simulink model "PIDControllerTest"  (R2025b)
settings: Solver=FixedStepAuto  StartTime=0.0  StopTime=inf  FixedStep=.01  RelTol=1e-3
settings Model: Creator=talles  LastModifiedBy=ajax

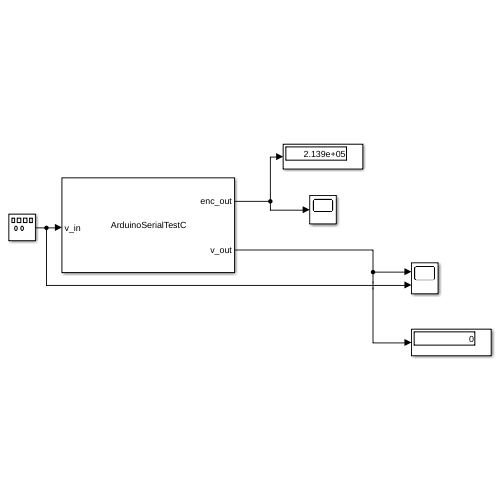
[thumbnail: Simulink's stored preview of the top-level diagram]
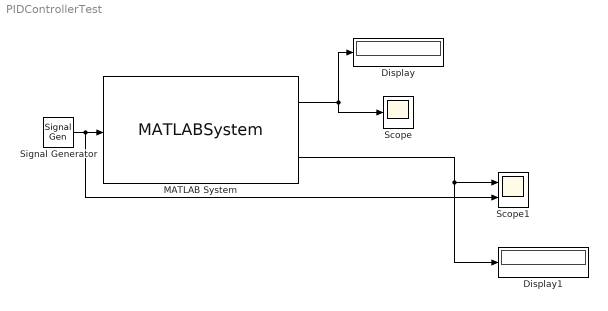
== system PIDControllerTest ==
  Display : Display
  Display1 : Display
  MATLAB System : MATLABSystem  System=ArduinoSerialTestC  COMPort=/dev/ttyACM0  BaudRate=115200  SimulateUsing=Interpreted execution
      mask Type: ArduinoSerialTestC
  Scope : Scope
      settings: ActiveDisplayYMinimum=-1.6860745042674926E+6  ActiveDisplayYMaximum=1.7659047746045869E+6
  Scope1 : Scope  NumInputPorts=2
      settings: ActiveDisplayYMinimum=-6.0034594760493682  ActiveDisplayYMaximum=14.706273819701902
  Signal Generator : SignalGenerator  WaveForm=square  Frequency=.5
  wires:
  MATLAB System/1 -> Display/1, Scope/1
  MATLAB System/2 -> Display1/1, Scope1/1
  Signal Generator/1 -> Scope1/2, MATLAB System/1
